simulink model "w3_warplab_agc"  (Simulink 7.7)
settings: Solver=ode45  StartTime=0.0  StopTime=1e4  RelTol=1e-3
PostLoadFcn:
  | w3_warplab_agc_init
InitFcn:
  | w3_warplab_agc_init
StartFcn:
  | w3_warplab_agc_init
undefined symbols (not defined in the file): gcbh, PHY_CONFIG_PKT_DET_CORR_THRESH, PHY_CONFIG_PKT_DET_ENERGY_THRESH, PHY_CONFIG_PKT_DET_MIN_DURR, xlBlockLoadCallback, xlGetNormalizedPeriod
libraries: xbsIndex_r4 x1039, xbsEDKLib_r4 x1, simulink x1
(part 1 of 7)
settings Model: Creator=murphpo  LastModifiedBy=mango
settings DebuggingCC: SolverPrmCheckMsg=none  InheritedTsInSrcMsg=none  FcnCallInpInsideContextMsg=Enable All  UnconnectedInputMsg=none  UnconnectedOutputMsg=none  UnconnectedLineMsg=none

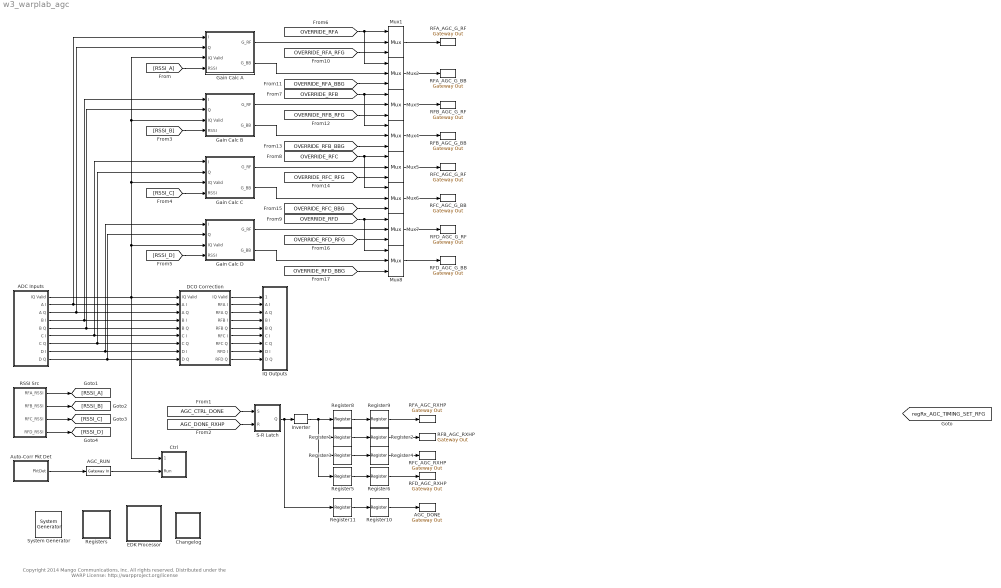
== system w3_warplab_agc ==
  note: Copyright 2014 Mango Communications, Inc. All rights reserved.
      |
      | Distributed under the WARP License:
      | http://warpproject.org/license
  " System Generator" : xbsIndex_r4/ System Generator  Tag=genX  SystemSampleTime=-1  xilinxfamily=virtex6  part=xc6vlx240t  speed=-2  package=ff1156  synthesis_tool=XST  clock_wrapper=Clock Enables  directory=./warplab_agc  proj_type=Project Navigator  Synth_file=XST Defaults  Impl_file=ISE Defaults  testbench=off  simulink_period=1  sysclk_period=10  dcm_input_clock_period=10  incr_netlist=off  trim_vbits=Everywhere in SubSystem  dbl_ovrd=According to Block Masks  core_generation=According to Block Masks  run_coregen=off  deprecated_control=off  eval_field=0  block_type=sysgen
  ADC Inputs : Subsystem
  AGC_DONE : xbsIndex_r4/Gateway Out  inherit_from_input=off  hdl_port=on  timing_constraint=None  locs_specified=off  LOCs={}  UseAsDAC=off  DACChannel='1'  block_type=gatewayout
  AGC_RUN : xbsIndex_r4/Gateway In  gui_display_data_type=Boolean  arith_type=Boolean  n_bits=16  bin_pt=14  preci_type=Single  exp_width=8  frac_width=24  quantization="Round  (unbiased: +/- Inf)"  overflow=Saturate  period=1  dbl_ovrd=off  timing_constraint=None  locs_specified=off  LOCs={}  UseAsADC=off  ADCChannel='1'  inherit_from_input=off  hdl_port=on  block_type=gatewayin
  Auto-Corr Pkt Det : Subsystem
  Changelog : Subsystem
  Ctrl : Subsystem
  DCO Correction : Subsystem
  EDK Processor : Subsystem  LoadFcn=xlBlockLoadCallback(gcbh);  mask(Xilinx EDK Processor Block){mode=EDK pcore generation, xmp=, MemVisToProc=<qt bgcolor="#FFFFFF"><div><img src="C:/Xilinx/14.4/ISE_DS/ISE/sysgen/data/images/registerplus.gif"> &lt;&lt;TIMING_RESET&gt;&gt;<br></div><div><img src="C:/Xilinx/14.4/ISE_DS/ISE/sysgen/data/images/registerplus.gif"> &lt;&lt;RSSI_PWR_CALIB&gt;&gt;<br></div><div><img src="C:/Xilinx/14.4/ISE_DS/ISE/sysgen/data/images/registerplus.gif"> &lt;&lt;IIR_COEF_B0&gt;&gt;<br></div><div><img src="C:/Xilinx/14.4/ISE_DS/ISE/sysgen/data/images/registerplus.gif"> &lt;&lt;IIR_COEF_A1&gt;&gt;<br></div><div><img src="C:/Xilinx/14.4/ISE_DS/ISE/sysgen/data/images/registerplus.gif"> &lt;&lt;RESET&gt;&gt;<br></div><div><img src="C:/Xilinx/14.4/ISE_DS/ISE/sysgen/data/images/registerplus.gif"> &lt;&lt;TIMING_AGC&gt;&gt;<br></div><div><img src="C:/Xilinx/14.4/ISE_DS/ISE/sysgen/data/images/registerplus.gif"> &lt;&lt;TARGET&gt;&gt;<br></div><div><img src="C:/Xilinx/14.4/ISE_DS/ISE/sysgen/data/images/registerplus.gif"> &lt;&lt;CONFIG&gt;&gt;<br></div><div><img src="C:/Xilinx/14.4/ISE_DS/ISE/sysgen/data/images/registerplus.gif"> &lt;&lt;RESET_MODE&gt;&gt;<br></div><div><img src="C:/Xilinx/14.4/ISE_DS/ISE/sysgen/data/images/registerplus.gif"> &lt;&lt;AGC_OVERRIDE&gt;&gt;<br></div><div><img src="C:/Xilinx/14.4/ISE_DS/ISE/sysgen/data/images/registerplus.gif"> &lt;&lt;RX_LENGTH&gt;&gt;<br></div><div><img src="C:/Xilinx/14.4/ISE_DS/ISE/sysgen/data/images/registerplus.gif"> &lt;&lt;TIMING_DCO&gt;&gt;<br></div></qt>, AvailableMemories=<empty>, portInterfaceTable={'exposed'=>[],'portdir'=>[],'portname'=>[],'shortname'=>[]}, bus_type_sgadvanced=, bus_type=AXI, baseaddr=0x80000000, baseaddr_lock_sgadvanced=, baseaddr_lock=off, dual_clock_sgadvanced=, dual_clock=on, reg_readback_sgadvanced=, reg_readback=on, ucf_file=, inheritDeviceType_sgadvanced=, inheritDeviceType=off, elf_file=, codebug_sgadvanced=, codebug=on, clock_name=plb, internalPortList={}, resetPolarity=0, memxtable={'mladdr'=>[0.00000000000000000,1.00000000000000000,2.00000000000000000,3.00000000000000000,4.00000000000000000,5.00000000000000000,6.00000000000000000,7.00000000000000000,8.00000000000000000,9.00000000000000000,10.00000000000000000,11.00000000000000000],'mlist'=>['w3_warplab_agc/Registers/From Register9','w3_warplab_agc/Registers/From Register8','w3_warplab_agc/Registers/From Register7','w3_warplab_agc/Registers/From Register6','w3_warplab_agc/Registers/From Register5','w3_warplab_agc/Registers/From Register4','w3_warplab_agc/Registers/From Register3','w3_warplab_agc/Registers/From Register2','w3_warplab_agc/Registers/From Register12','w3_warplab_agc/Registers/From Register11','w3_warplab_agc/Registers/From Register10','w3_warplab_agc/Registers/From Register1'],'mlname'=>['\\'TIMING_RESET\\'','\\'RSSI_PWR_CALIB\\'','\\'IIR_COEF_B0\\'','\\'IIR_COEF_A1\\'','\\'RESET\\'','\\'TIMING_AGC\\'','\\'TARGET\\'','\\'CONFIG\\'','\\'RESET_MODE\\'','\\'AGC_OVERRIDE\\'','\\'RX_LENGTH\\'','\\'TIMING_DCO\\''],'mlstate'=>[0.00000000000000000,0.00000000000000000,0.00000000000000000,0.00000000000000000,0.00000000000000000,0.00000000000000000,0.00000000000000000,0.00000000000000000,0.00000000000000000,0.00000000000000000,0.00000000000000000,0.00000000000000000]}, procinfo={}, memmapdirty=off, blockname=, xpsintstyle=default, has_advanced_control=0, sggui_pos=-1,-1,-1,-1, block_type=edkprocessor, block_version=2.7, sg_icon_stat=62,64,-1,-1,white,blue,0,07734,right,,[ ],[ ], sg_mask_display=|, sg_list_contents={'table'=>{'AvailableMemories'=>'popup(<empty>)'}}, sg_blockgui_xml=}
      mask sg_mask_display=|
      | fprintf('','COMMENT: begin icon graphics');
      | patch([0 62 62 0 0 ],[0 0 64 64 0 ],[0.77 0.82 0.91 ]);
      | plot([0 62 62 0 0 ],[0 0 64 64 0 ]);
      | patch([13.2 24.76 32.76 40.76 48.76 32.76 21.2 13.2 ],[40.88 40.88 48.88 40.88 48.88 48.88 48.88 40.88 ],[1 1 1 ]);
      | patch([21.2 32.76 24.76 13.2 21.2 ],[32.88 32.88 40.88 40.88 32.88 ],[0.931 0.946 0.973 ]);
      | patch([13.2 24.76 32.76 21.2 13.2 ],[24.88 24.88 32.88 32.88 24.88 ],[1 1 1 ]);
      | patch([21.2 48.76 40.76 32.76 24.76 13.2 21.2 ],[16.88 16.88 24.88 16.88 24.88 24.88 16.88 ],[0.931 0.946 0.973 ]);
      | fprintf('','COMMENT: end icon graphics');
      | fprintf('','COMMENT: begin icon text');
      | fprintf('','COMMENT: end icon text');
      mask prompts: mode "Configure Processor for"; xmp "XPS Project"; MemVisToProc ""; AvailableMemories "Available Memories"; portInterfaceTable ""; bus_type_sgadvanced ""; bus_type "Bus Type"; baseaddr "Base Address"; baseaddr_lock_sgadvanced ""; baseaddr_lock "Lock"; dual_clock_sgadvanced ""; dual_clock "Dual Clocks"; reg_readback_sgadvanced ""; reg_readback "Register Read-Back"; ucf_file "Constraint File"; inheritDeviceType_sgadvanced ""; inheritDeviceType "Inherit Device Type"; elf_file "Initial Program"; codebug_sgadvanced ""; codebug "Enable Co-Debug with Xilinx SDK (Beta)"; clock_name ""; internalPortList ""; resetPolarity ""; memxtable ""; procinfo ""; memmapdirty ""; blockname ""; xpsintstyle ""; has_advanced_control ""; sggui_pos ""; block_type ""; block_version ""; sg_icon_stat ""; sg_mask_display ""; sg_list_contents ""; sg_blockgui_xml ""
      mask help: Xilinx EDK Processor
      mask init:
      | try
      |   tmp_gcb = gcb;
      |   tmp_gcbh = gcbh;
      |   if (strcmp('SysGenIndex',get_param(bdroot(tmp_gcbh),'tag')) && ~isempty(regexp(bdroot(tmp_gcb), '^xbs', 'once')))
      |     return;
      |   end;
      |   xlMungeMaskParams;
      | 
      |   block_type='edkprocessor';
      | 
      |   serialized_declarations = '{''block_type''=>''String''}';
      |   xledkprocessor_init();
      |   ptable_ = xlblockprep(get_param(tmp_gcb, 'MaskWSVariables'));
      |   try
      |     xlBlockMoveCallback(tmp_gcbh);
      |   catch 
      |      clear global xl_updateicon_recursion_guard;
      |   end;
      | catch
      |   global dbgsysgen;
      |   if(~isempty(dbgsysgen) && dbgsysgen)
      |     e = regexprep(lasterr, '\n', '\nError: ');
      |     disp(['Error: While running MaskInit code on block ' tmp_gcb ': ' e]);
      |     error(e);
      |   end
      | end
      settings: CopyFcn=xlProcBlockCopyCallback(gcbh);xlBlockMoveCallback(gcbh);  DeleteFcn=xlDestroyGui(gcbh);  ModelCloseFcn=xlDestroyGui(gcbh);  PreSaveFcn=xlBlockPreSaveCallback(gcbh);  PostSaveFcn=xlBlockPostSaveCallback(gcbh);  DestroyFcn=xlDestroyGui(gcbh);  OpenFcn=bh=gcbh;xlProcBlockCallbacks('populatesharedmemorylistbox',bh);xlOpenGui(bh, 'edkprocessor_gui.xml', @xlProcBlockEnablement, @xlProcBlockAction);  CloseFcn=xlDestroyGui(gcbh);  MoveFcn=xlBlockMoveCallback(gcbh);
      mask Help: eval('');xlDoc('-book','sysgen','-topic','EDK_Processor');
      mask StyleString: popup(EDK pcore generation|HDL netlisting),edit,edit,edit,edit,edit,popup(AXI|PLB),edit,edit,checkbox,edit,checkbox,edit,checkbox,edit,edit,checkbox,edit,edit,checkbox,edit,edit,edit,edit,edit,edit,edit,edit,edit,edit,edit,edit,edit,edit,edit,edit
      mask Display:
      | fprintf('','COMMENT: begin icon graphics');
      | patch([0 62 62 0 0 ],[0 0 64 64 0 ],[0.77 0.82 0.91 ]);
      | plot([0 62 62 0 0 ],[0 0 64 64 0 ]);
      | patch([13.2 24.76 32.76 40.76 48.76 32.76 21.2 13.2 ],[40.88 40.88 48.88 40.88 48.88 48.88 48.88 40.88 ],[1 1 1 ]);
      | patch([21.2 32.76 24.76 13.2 21.2 ],[32.88 32.88 40.88 40.88 32.88 ],[0.931 0.946 0.973 ]);
      | patch([13.2 24.76 32.76 21.2 13.2 ],[24.88 24.88 32.88 32.88 24.88 ],[1 1 1 ]);
      | patch([21.2 48.76 40.76 32.76 24.76 13.2 21.2 ],[16.88 16.88 24.88 16.88 24.88 24.88 16.88 ],[0.931 0.946 0.973 ]);
      | fprintf('','COMMENT: end icon graphics');
      | fprintf('','COMMENT: begin icon text');
      | disp('');
      | 
      | fprintf('','COMMENT: end icon text');
  Gain Calc A : Subsystem
  Gain Calc B : Subsystem
  Gain Calc C : Subsystem
  Gain Calc D : Subsystem
  IQ Outputs : Subsystem
  Inverter : xbsIndex_r4/Inverter  en=off  latency=0  dbl_ovrd=off  block_type=inv
      settings: xl_area=[0 0 0 0 0 0 0]  block_version=VER_STRING_GOES_HERE
  Mux{1..8} (8 alike) : xbsIndex_r4/Mux  inputs=2  en=off  latency=0  precision=Full  arith_type=Unsigned  n_bits=16  bin_pt=14  quantization=Truncate  overflow=Wrap  dbl_ovrd=off  block_type=mux
  RFA_AGC_G_BB : xbsIndex_r4/Gateway Out  inherit_from_input=off  hdl_port=on  timing_constraint=None  locs_specified=off  LOCs={}  UseAsDAC=off  DACChannel='1'  block_type=gatewayout
  RFA_AGC_G_RF : xbsIndex_r4/Gateway Out  inherit_from_input=off  hdl_port=on  timing_constraint=None  locs_specified=off  LOCs={}  UseAsDAC=off  DACChannel='1'  block_type=gatewayout
  RFA_AGC_RXHP : xbsIndex_r4/Gateway Out  inherit_from_input=off  hdl_port=on  timing_constraint=None  locs_specified=off  LOCs={}  UseAsDAC=off  DACChannel='1'  block_type=gatewayout
  RFB_AGC_G_BB : xbsIndex_r4/Gateway Out  inherit_from_input=off  hdl_port=on  timing_constraint=None  locs_specified=off  LOCs={}  UseAsDAC=off  DACChannel='1'  block_type=gatewayout
  RFB_AGC_G_RF : xbsIndex_r4/Gateway Out  inherit_from_input=off  hdl_port=on  timing_constraint=None  locs_specified=off  LOCs={}  UseAsDAC=off  DACChannel='1'  block_type=gatewayout
  RFB_AGC_RXHP : xbsIndex_r4/Gateway Out  inherit_from_input=off  hdl_port=on  timing_constraint=None  locs_specified=off  LOCs={}  UseAsDAC=off  DACChannel='1'  block_type=gatewayout
  RFC_AGC_G_BB : xbsIndex_r4/Gateway Out  inherit_from_input=off  hdl_port=on  timing_constraint=None  locs_specified=off  LOCs={}  UseAsDAC=off  DACChannel='1'  block_type=gatewayout
  RFC_AGC_G_RF : xbsIndex_r4/Gateway Out  inherit_from_input=off  hdl_port=on  timing_constraint=None  locs_specified=off  LOCs={}  UseAsDAC=off  DACChannel='1'  block_type=gatewayout
  RFC_AGC_RXHP : xbsIndex_r4/Gateway Out  inherit_from_input=off  hdl_port=on  timing_constraint=None  locs_specified=off  LOCs={}  UseAsDAC=off  DACChannel='1'  block_type=gatewayout
  RFD_AGC_G_BB : xbsIndex_r4/Gateway Out  inherit_from_input=off  hdl_port=on  timing_constraint=None  locs_specified=off  LOCs={}  UseAsDAC=off  DACChannel='1'  block_type=gatewayout
  RFD_AGC_G_RF : xbsIndex_r4/Gateway Out  inherit_from_input=off  hdl_port=on  timing_constraint=None  locs_specified=off  LOCs={}  UseAsDAC=off  DACChannel='1'  block_type=gatewayout
  RFD_AGC_RXHP : xbsIndex_r4/Gateway Out  inherit_from_input=off  hdl_port=on  timing_constraint=None  locs_specified=off  LOCs={}  UseAsDAC=off  DACChannel='1'  block_type=gatewayout
  RSSI Src : Subsystem
  Register{1..6,8..11} (10 alike) : xbsIndex_r4/Register  init=0  rst=off  en=off  dbl_ovrd=off  block_type=register
  Registers : Subsystem
  S-R Latch : Subsystem
  tag scope: regRx_AGC_TIMING_SET_RFG=global
  wires:
  AGC_RUN/1 -> Ctrl/2(Run)
  [AGC_CTRL_DONE] -> S-R Latch/1(S)
  [AGC_DONE_RXHP] -> S-R Latch/2(R)
  S-R Latch/1(Q) -> Inverter/1, Register11/1
  Register8/1 -> Register9/1
  Register9/1 -> RFA_AGC_RXHP/1
  Inverter/1 -> Register8/1, Register1/1, Register3/1, Register5/1
  Register10/1 -> AGC_DONE/1
  Register11/1 -> Register10/1
  Register1/1 -> Register2/1
  Register2/1 -> RFB_AGC_RXHP/1
  ADC Inputs/1(IQ Valid) -> DCO Correction/1(IQ Valid), Gain Calc A/3(IQ Valid), Gain Calc B/3(IQ Valid), Gain Calc C/3(IQ Valid), Gain Calc D/3(IQ Valid), Ctrl/1(IQ Valid)
  ADC Inputs/2(A I) -> DCO Correction/2(A I), Gain Calc A/1(I)
  ADC Inputs/3(A Q) -> DCO Correction/3(A Q), Gain Calc A/2(Q)
  ADC Inputs/4(B I) -> DCO Correction/4(B I), Gain Calc B/1(I)
  ADC Inputs/5(B Q) -> DCO Correction/5(B Q), Gain Calc B/2(Q)
  ADC Inputs/6(C I) -> DCO Correction/6(C I), Gain Calc C/1(I)
  ADC Inputs/7(C Q) -> DCO Correction/7(C Q), Gain Calc C/2(Q)
  ADC Inputs/8(D I) -> DCO Correction/8(D I), Gain Calc D/1(I)
  ADC Inputs/9(D Q) -> DCO Correction/9(D Q), Gain Calc D/2(Q)
  DCO Correction/1(" IQ Valid") -> IQ Outputs/1(IQ Valid)
  DCO Correction/2(" RFA I") -> IQ Outputs/2(A I)
  DCO Correction/3(" RFA Q") -> IQ Outputs/3(A Q)
  DCO Correction/4(RFB I) -> IQ Outputs/4(B I)
  DCO Correction/5(RFB Q) -> IQ Outputs/5(B Q)
  DCO Correction/6(RFC I) -> IQ Outputs/6(C I)
  DCO Correction/7(RFC Q) -> IQ Outputs/7(C Q)
  DCO Correction/8(RFD I) -> IQ Outputs/8(D I)
  DCO Correction/9(RFD Q) -> IQ Outputs/9(D Q)
  RSSI Src/1(" RFA_RSSI") -> [RSSI_A]
  RSSI Src/2(" RFB_RSSI") -> [RSSI_B]
  [RSSI_A] -> Gain Calc A/4(RSSI)
  [RSSI_B] -> Gain Calc B/4(RSSI)
  [RSSI_C] -> Gain Calc C/4(RSSI)
  [RSSI_D] -> Gain Calc D/4(RSSI)
  Register3/1 -> Register4/1
  Register4/1 -> RFC_AGC_RXHP/1
  Register5/1 -> Register6/1
  Register6/1 -> RFD_AGC_RXHP/1
  RSSI Src/3(" RFC_RSSI") -> [RSSI_C]
  RSSI Src/4(" RFD_RSSI") -> [RSSI_D]
  [OVERRIDE_RFA] -> Mux1/1, Mux2/1
  Mux1/1 -> RFA_AGC_G_RF/1
  Mux2/1 -> RFA_AGC_G_BB/1
  Mux3/1 -> RFB_AGC_G_RF/1
  Mux4/1 -> RFB_AGC_G_BB/1
  Mux5/1 -> RFC_AGC_G_RF/1
  Mux6/1 -> RFC_AGC_G_BB/1
  Mux7/1 -> RFD_AGC_G_RF/1
  Mux8/1 -> RFD_AGC_G_BB/1
  [OVERRIDE_RFB] -> Mux3/1, Mux4/1
  [OVERRIDE_RFA_RFG] -> Mux1/3
  [OVERRIDE_RFA_BBG] -> Mux2/3
  Gain Calc A/1(G_RF) -> Mux1/2
  Gain Calc A/2(G_BB) -> Mux2/2
  Gain Calc B/1(G_RF) -> Mux3/2
  [OVERRIDE_RFB_RFG] -> Mux3/3
  Gain Calc B/2(G_BB) -> Mux4/2
  [OVERRIDE_RFB_BBG] -> Mux4/3
  [OVERRIDE_RFC] -> Mux5/1, Mux6/1
  [OVERRIDE_RFD] -> Mux7/1, Mux8/1
  Gain Calc C/1(G_RF) -> Mux5/2
  Gain Calc C/2(G_BB) -> Mux6/2
  Gain Calc D/1(G_RF) -> Mux7/2
  Gain Calc D/2(G_BB) -> Mux8/2
  [OVERRIDE_RFC_RFG] -> Mux5/3
  [OVERRIDE_RFC_BBG] -> Mux6/3
  [OVERRIDE_RFD_RFG] -> Mux7/3
  [OVERRIDE_RFD_BBG] -> Mux8/3
  Auto-Corr Pkt Det/1(PktDet) -> AGC_RUN/1

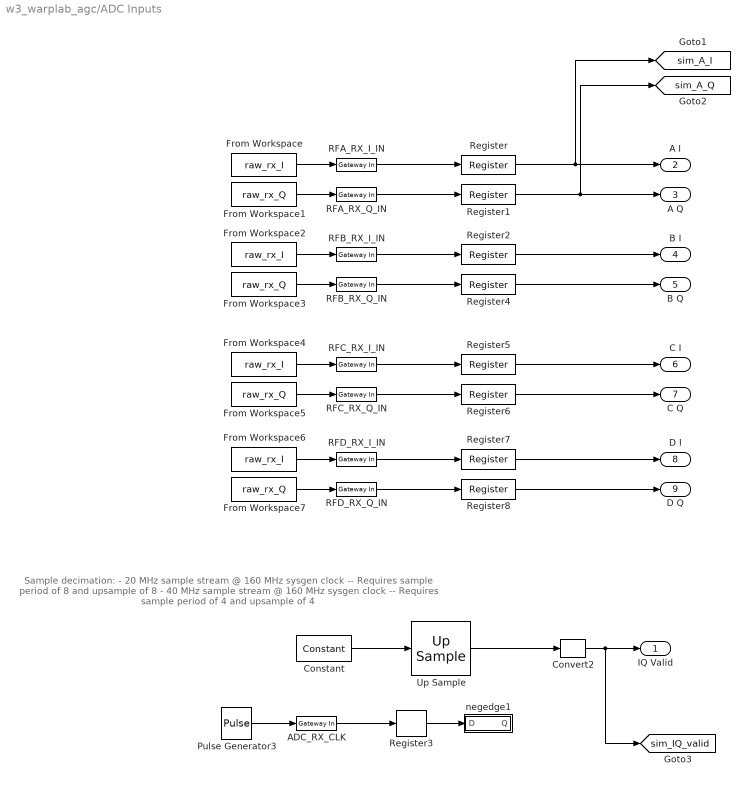
== system w3_warplab_agc/ADC Inputs ==
  note: Sample decimation:
      |   - 20 MHz sample stream @ 160 MHz sysgen clock -- Requires sample period of 8 and upsample of 8
      |   - 40 MHz sample stream @ 160 MHz sysgen clock -- Requires sample period of 4 and upsample of 4
  ADC_RX_CLK : xbsIndex_r4/Gateway In  gui_display_data_type=Boolean  arith_type=Boolean  n_bits=1  bin_pt=0  preci_type=Single  exp_width=8  frac_width=24  quantization="Round  (unbiased: +/- Inf)"  overflow=Saturate  period=1  dbl_ovrd=off  timing_constraint=None  locs_specified=off  LOCs={}  UseAsADC=off  ADCChannel='1'  inherit_from_input=off  hdl_port=on  block_type=gatewayin
  Constant : xbsIndex_r4/Constant  const=1  gui_display_data_type=Boolean  arith_type=Boolean  n_bits=16  bin_pt=14  preci_type=Single  exp_width=8  frac_width=24  explicit_period=on  period=4  equ=P=C  opselect=C  inp2=PCIN>>17  opr=+  inp1=P  carry=CIN  dbl_ovrd=off  block_type=constant
  Convert2 : xbsIndex_r4/Convert  gui_display_data_type=Boolean  arith_type=Boolean  n_bits=1  bin_pt=0  float_type=Single  exp_bits=8  fraction_bits=24  quantization=Truncate  overflow=Wrap  en=off  latency=0  dbl_ovrd=off  pipeline=off  block_type=convert
  From Workspace{,2,4,6} (4 alike) : FromWorkspace  VariableName=raw_rx_I  SampleTime=4  Interpolate=off  OutputAfterFinalValue=Setting to zero
  From Workspace{1,3,5,7} (4 alike) : FromWorkspace  VariableName=raw_rx_Q  SampleTime=4  Interpolate=off  OutputAfterFinalValue=Setting to zero
  Pulse Generator3 : DiscretePulseGenerator  Period=8  PulseWidth=4
  RFA_RX_I_IN : xbsIndex_r4/Gateway In  gui_display_data_type=Fixed-point  arith_type="Signed  (2's comp)"  n_bits=12  bin_pt=11  preci_type=Single  exp_width=8  frac_width=24  quantization="Round  (unbiased: +/- Inf)"  overflow=Saturate  period=1  dbl_ovrd=off  timing_constraint=None  locs_specified=off  LOCs={}  UseAsADC=off  ADCChannel='1'  inherit_from_input=off  hdl_port=on  block_type=gatewayin
  RFA_RX_Q_IN : xbsIndex_r4/Gateway In  gui_display_data_type=Fixed-point  arith_type="Signed  (2's comp)"  n_bits=12  bin_pt=11  preci_type=Single  exp_width=8  frac_width=24  quantization="Round  (unbiased: +/- Inf)"  overflow=Saturate  period=1  dbl_ovrd=off  timing_constraint=None  locs_specified=off  LOCs={}  UseAsADC=off  ADCChannel='1'  inherit_from_input=off  hdl_port=on  block_type=gatewayin
  RFB_RX_I_IN : xbsIndex_r4/Gateway In  gui_display_data_type=Fixed-point  arith_type="Signed  (2's comp)"  n_bits=12  bin_pt=11  preci_type=Single  exp_width=8  frac_width=24  quantization="Round  (unbiased: +/- Inf)"  overflow=Saturate  period=1  dbl_ovrd=off  timing_constraint=None  locs_specified=off  LOCs={}  UseAsADC=off  ADCChannel='1'  inherit_from_input=off  hdl_port=on  block_type=gatewayin
  RFB_RX_Q_IN : xbsIndex_r4/Gateway In  gui_display_data_type=Fixed-point  arith_type="Signed  (2's comp)"  n_bits=12  bin_pt=11  preci_type=Single  exp_width=8  frac_width=24  quantization="Round  (unbiased: +/- Inf)"  overflow=Saturate  period=1  dbl_ovrd=off  timing_constraint=None  locs_specified=off  LOCs={}  UseAsADC=off  ADCChannel='1'  inherit_from_input=off  hdl_port=on  block_type=gatewayin
  RFC_RX_I_IN : xbsIndex_r4/Gateway In  gui_display_data_type=Fixed-point  arith_type="Signed  (2's comp)"  n_bits=12  bin_pt=11  preci_type=Single  exp_width=8  frac_width=24  quantization="Round  (unbiased: +/- Inf)"  overflow=Saturate  period=1  dbl_ovrd=off  timing_constraint=None  locs_specified=off  LOCs={}  UseAsADC=off  ADCChannel='1'  inherit_from_input=off  hdl_port=on  block_type=gatewayin
  RFC_RX_Q_IN : xbsIndex_r4/Gateway In  gui_display_data_type=Fixed-point  arith_type="Signed  (2's comp)"  n_bits=12  bin_pt=11  preci_type=Single  exp_width=8  frac_width=24  quantization="Round  (unbiased: +/- Inf)"  overflow=Saturate  period=1  dbl_ovrd=off  timing_constraint=None  locs_specified=off  LOCs={}  UseAsADC=off  ADCChannel='1'  inherit_from_input=off  hdl_port=on  block_type=gatewayin
  RFD_RX_I_IN : xbsIndex_r4/Gateway In  gui_display_data_type=Fixed-point  arith_type="Signed  (2's comp)"  n_bits=12  bin_pt=11  preci_type=Single  exp_width=8  frac_width=24  quantization="Round  (unbiased: +/- Inf)"  overflow=Saturate  period=1  dbl_ovrd=off  timing_constraint=None  locs_specified=off  LOCs={}  UseAsADC=off  ADCChannel='1'  inherit_from_input=off  hdl_port=on  block_type=gatewayin
  RFD_RX_Q_IN : xbsIndex_r4/Gateway In  gui_display_data_type=Fixed-point  arith_type="Signed  (2's comp)"  n_bits=12  bin_pt=11  preci_type=Single  exp_width=8  frac_width=24  quantization="Round  (unbiased: +/- Inf)"  overflow=Saturate  period=1  dbl_ovrd=off  timing_constraint=None  locs_specified=off  LOCs={}  UseAsADC=off  ADCChannel='1'  inherit_from_input=off  hdl_port=on  block_type=gatewayin
  Register{,1..8} (9 alike) : xbsIndex_r4/Register  init=0  rst=off  en=off  dbl_ovrd=off  block_type=register
  Up Sample : xbsIndex_r4/Up Sample  sample_ratio=4  copy_samples=off  en=off  latency=0  dbl_ovrd=off  block_type=usamp
  negedge1 : Subsystem
  IQ Valid : Outport
  A I : Outport  Port=2
  A Q : Outport  Port=3
  B I : Outport  Port=4
  B Q : Outport  Port=5
  C I : Outport  Port=6
  C Q : Outport  Port=7
  D I : Outport  Port=8
  D Q : Outport  Port=9
  tag scope: sim_A_I=global, sim_A_Q=global, sim_IQ_valid=global
  wires:
  From Workspace/1 -> RFA_RX_I_IN/1
  From Workspace1/1 -> RFA_RX_Q_IN/1
  RFA_RX_I_IN/1 -> Register/1
  RFA_RX_Q_IN/1 -> Register1/1
  From Workspace2/1 -> RFB_RX_I_IN/1
  From Workspace3/1 -> RFB_RX_Q_IN/1
  RFB_RX_I_IN/1 -> Register2/1
  RFB_RX_Q_IN/1 -> Register4/1
  Up Sample/1 -> Convert2/1
  Register3/1 -> negedge1/1(D)
  ADC_RX_CLK/1 -> Register3/1
  Pulse Generator3/1 -> ADC_RX_CLK/1
  Convert2/1 -> IQ Valid/1, [sim_IQ_valid]
  RFC_RX_I_IN/1 -> Register5/1
  RFC_RX_Q_IN/1 -> Register6/1
  RFD_RX_I_IN/1 -> Register7/1
  RFD_RX_Q_IN/1 -> Register8/1
  Constant/1 -> Up Sample/1
  From Workspace4/1 -> RFC_RX_I_IN/1
  From Workspace5/1 -> RFC_RX_Q_IN/1
  From Workspace6/1 -> RFD_RX_I_IN/1
  From Workspace7/1 -> RFD_RX_Q_IN/1
  Register/1 -> A I/1, [sim_A_I]
  Register1/1 -> A Q/1, [sim_A_Q]
  Register2/1 -> B I/1
  Register4/1 -> B Q/1
  Register5/1 -> C I/1
  Register6/1 -> C Q/1
  Register7/1 -> D I/1
  Register8/1 -> D Q/1

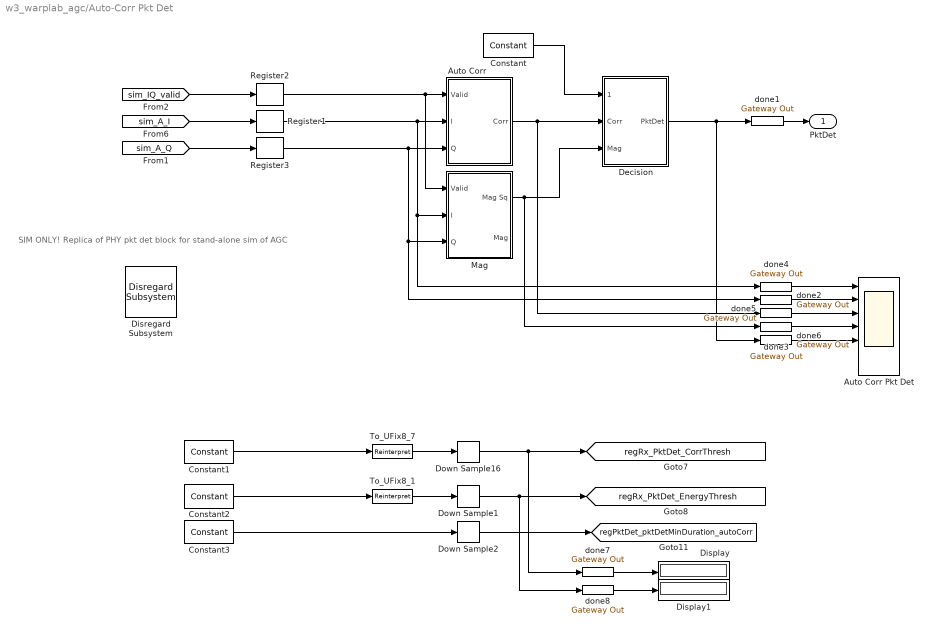
== system w3_warplab_agc/Auto-Corr Pkt Det ==
  note: SIM ONLY!
      | Replica of PHY pkt det block
      | for stand-alone sim of AGC
  Auto Corr : Subsystem
  Auto Corr Pkt Det : Scope  NumInputPorts=7
      settings: TimeRange=10000  YMin=-0.4~-0.4~-0.2~-0.2~-0.01~-1~0  YMax=0.4~0.4~0.2~0.2~0.02~1~0.8  SaveName=ScopeData28
  Constant : xbsIndex_r4/Constant  const=0  gui_display_data_type=Boolean  arith_type=Boolean  n_bits=16  bin_pt=14  preci_type=Single  exp_width=8  frac_width=24  explicit_period=off  period=1  equ=P=C  opselect=C  inp2=PCIN>>17  opr=+  inp1=P  carry=CIN  dbl_ovrd=off  block_type=constant
  Constant1 : xbsIndex_r4/Constant  const=PHY_CONFIG_PKT_DET_CORR_THRESH  gui_display_data_type=Fixed-point  arith_type=Unsigned  n_bits=8  bin_pt=0  preci_type=Single  exp_width=8  frac_width=24  explicit_period=on  period=1  equ=P=C  opselect=C  inp2=PCIN>>17  opr=+  inp1=P  carry=CIN  dbl_ovrd=off  block_type=constant
  Constant2 : xbsIndex_r4/Constant  const=PHY_CONFIG_PKT_DET_ENERGY_THRESH  gui_display_data_type=Fixed-point  arith_type=Unsigned  n_bits=16  bin_pt=0  preci_type=Single  exp_width=8  frac_width=24  explicit_period=on  period=1  equ=P=C  opselect=C  inp2=PCIN>>17  opr=+  inp1=P  carry=CIN  dbl_ovrd=off  block_type=constant
  Constant3 : xbsIndex_r4/Constant  const=PHY_CONFIG_PKT_DET_MIN_DURR  gui_display_data_type=Fixed-point  arith_type=Unsigned  n_bits=6  bin_pt=0  preci_type=Single  exp_width=8  frac_width=24  explicit_period=on  period=1  equ=P=C  opselect=C  inp2=PCIN>>17  opr=+  inp1=P  carry=CIN  dbl_ovrd=off  block_type=constant
  Decision : Subsystem
  Display : Display
  Display1 : Display
  Disregard Subsystem : xbsIndex_r4/Disregard Subsystem  Tag=discardX  block_type=disregard
  Down Sample1 : xbsIndex_r4/Down Sample  sample_ratio=8  sample_phase="Last Value of Frame  (most efficient)"  en=off  latency=1  dbl_ovrd=off  block_type=dsamp
      settings: block_version=VER_STRING_GOES_HERE
  Down Sample16 : xbsIndex_r4/Down Sample  sample_ratio=8  sample_phase="Last Value of Frame  (most efficient)"  en=off  latency=1  dbl_ovrd=off  block_type=dsamp
      settings: block_version=VER_STRING_GOES_HERE
  Down Sample2 : xbsIndex_r4/Down Sample  sample_ratio=8  sample_phase="Last Value of Frame  (most efficient)"  en=off  latency=1  dbl_ovrd=off  block_type=dsamp
      settings: block_version=VER_STRING_GOES_HERE
  Mag : Subsystem
  Register1 : xbsIndex_r4/Register  init=0  rst=off  en=off  dbl_ovrd=off  block_type=register
  Register2 : xbsIndex_r4/Register  init=0  rst=off  en=off  dbl_ovrd=off  block_type=register
  Register3 : xbsIndex_r4/Register  init=0  rst=off  en=off  dbl_ovrd=off  block_type=register
  To_UFix8_1 : xbsIndex_r4/Reinterpret  force_arith_type=on  arith_type=Unsigned  force_bin_pt=on  bin_pt=8  block_type=cast
      settings: infoedit="Changes type of samples without altering their binary representation.<P><P>Hardware notes: In hardware this block costs nothing.<P><P>Example:  Suppose the input is 6 bits wide, signed, with 2 fractional bits, and the output is forced to unsigned with 0 fractional bits.  Then an input of -2.0 (1110.00 in binary 2's complement) becomes an output of 56 (111000 in binary)."  block_version=VER_STRING_GOES_HERE
  To_UFix8_7 : xbsIndex_r4/Reinterpret  force_arith_type=on  arith_type=Unsigned  force_bin_pt=on  bin_pt=7  block_type=cast
      settings: infoedit="Changes type of samples without altering their binary representation.<P><P>Hardware notes: In hardware this block costs nothing.<P><P>Example:  Suppose the input is 6 bits wide, signed, with 2 fractional bits, and the output is forced to unsigned with 0 fractional bits.  Then an input of -2.0 (1110.00 in binary 2's complement) becomes an output of 56 (111000 in binary)."  block_version=VER_STRING_GOES_HERE
  done{1..8} (8 alike) : xbsIndex_r4/Gateway Out  inherit_from_input=off  hdl_port=off  timing_constraint=None  locs_specified=off  LOCs={}  UseAsDAC=off  DACChannel='1'  block_type=gatewayout
      settings: infoedit="Gateway out block.  Converts Xilinx fixed point inputs into ouputs of type Simulink integer, double, or fixed point.<P><P>Hardware notes:  In hardware these blocks become top level output ports or are discarded, depending on how they are configured."  xl_area=[0 0 0 0 1 0 0]  block_version=VER_STRING_GOES_HERE
  PktDet : Outport
  tag scope: regPktDet_pktDetMinDuration_autoCorr=global, regRx_PktDet_CorrThresh=global, regRx_PktDet_EnergyThresh=global
  wires:
  done4/1 -> Auto Corr Pkt Det/1
  [sim_A_Q] -> Register3/1
  [sim_A_I] -> Register1/1
  [sim_IQ_valid] -> Register2/1
  done2/1 -> Auto Corr Pkt Det/2
  done6/1 -> Auto Corr Pkt Det/5
  Register1/1 -> Auto Corr/2(I), Mag/2(I), done4/1
  Register3/1 -> Auto Corr/3(Q), Mag/3(Q), done2/1
  Register2/1 -> Auto Corr/1(Valid), Mag/1(Valid)
  Auto Corr/1(Corr) -> Decision/2(Corr), done5/1
  Mag/1(Mag Sq) -> Decision/3(Mag), done3/1
  done5/1 -> Auto Corr Pkt Det/3
  done3/1 -> Auto Corr Pkt Det/4
  Decision/1(PktDet) -> done6/1, done1/1
  Constant/1 -> Decision/1(PktDet Reset)
  done1/1 -> PktDet/1
  To_UFix8_7/1 -> Down Sample16/1
  To_UFix8_1/1 -> Down Sample1/1
  Down Sample16/1 -> [regRx_PktDet_CorrThresh], done7/1
  Down Sample1/1 -> [regRx_PktDet_EnergyThresh], done8/1
  Constant3/1 -> Down Sample2/1
  Down Sample2/1 -> [regPktDet_pktDetMinDuration_autoCorr]
  Constant1/1 -> To_UFix8_7/1
  Constant2/1 -> To_UFix8_1/1
  done7/1 -> Display/1
  done8/1 -> Display1/1

== system w3_warplab_agc/Changelog ==
  note: 3.00.a:
      | - Initial release.  Modified from 802.11 Reference Design
  note: 3.01.a:
      | - Fixed bug in handover between DCO and IIR HPF outputs.

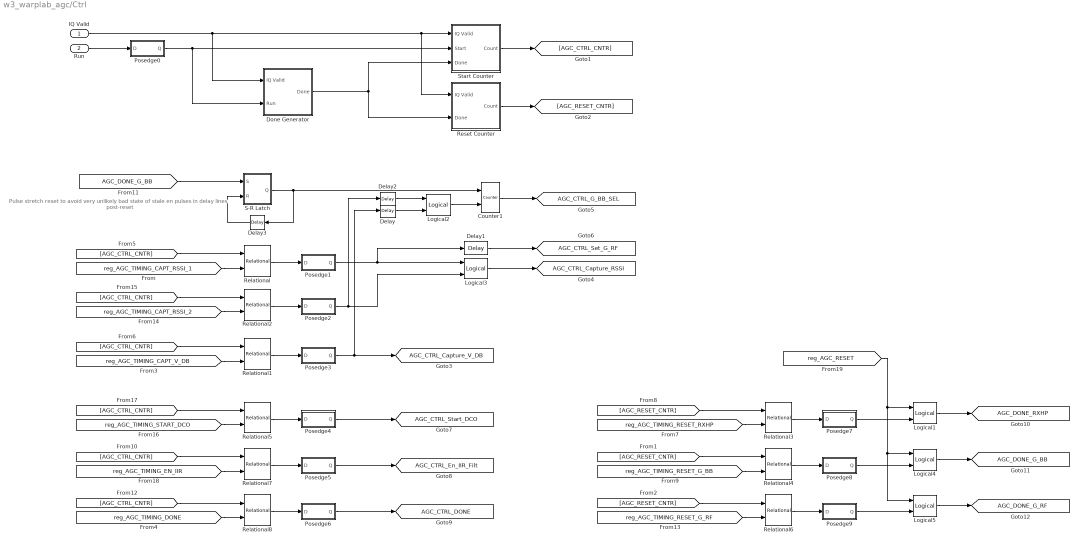
== system w3_warplab_agc/Ctrl ==
  note: Pulse stretch reset to avoid very
      | unlikely bad state of stale
      | en pulses in delay lines
      | post-reset
  IQ Valid : Inport
  Run : Inport  Port=2
  Counter1 : xbsIndex_r4/Counter  cnt_type=Free Running  cnt_to=1023  operation=Up  start_count=0  cnt_by_val=1  arith_type=Unsigned  n_bits=2  bin_pt=0  load_pin=off  rst=on  en=on  explicit_period=off  period=1  dbl_ovrd=off  use_behavioral_HDL=off  implementation=Fabric  block_type=counter
  Delay : xbsIndex_r4/Delay  rst=off  infoeditControl=Selection of Reset will increase slice count due to use of real FFs and instead of SRLs  en=off  latency=2  dbl_ovrd=off  reg_retiming=off  block_type=delay
      settings: xl_area=[7 14 0 14 0 0 0]  block_version=VER_STRING_GOES_HERE
  Delay1 : xbsIndex_r4/Delay  rst=off  infoeditControl=Selection of Reset will increase slice count due to use of real FFs and instead of SRLs  en=off  latency=5  dbl_ovrd=off  reg_retiming=off  block_type=delay
      settings: xl_area=[7 14 0 14 0 0 0]  block_version=VER_STRING_GOES_HERE
  Delay2 : xbsIndex_r4/Delay  rst=off  infoeditControl=Selection of Reset will increase slice count due to use of real FFs and instead of SRLs  en=off  latency=6  dbl_ovrd=off  reg_retiming=off  block_type=delay
      settings: xl_area=[7 14 0 14 0 0 0]  block_version=VER_STRING_GOES_HERE
  Delay3 : xbsIndex_r4/Delay  rst=off  infoeditControl=Selection of Reset will increase slice count due to use of real FFs and instead of SRLs  en=off  latency=6  dbl_ovrd=off  reg_retiming=off  block_type=delay
      settings: xl_area=[7 14 0 14 0 0 0]  block_version=VER_STRING_GOES_HERE
  Done Generator : Subsystem
  Logical{1..5} (5 alike) : xbsIndex_r4/Logical  logical_function=OR  inputs=2  en=off  latency=0  precision=Full  arith_type=Unsigned  n_bits=16  bin_pt=0  align_bp=on  dbl_ovrd=off  block_type=logical
  Posedge0 : Subsystem
  Posedge1 : Subsystem
  Posedge2 : Subsystem
  Posedge3 : Subsystem
  Posedge4 : Subsystem
  Posedge5 : Subsystem
  Posedge6 : Subsystem
  Posedge7 : Subsystem
  Posedge8 : Subsystem
  Posedge9 : Subsystem
  Relational{,1..8} (9 alike) : xbsIndex_r4/Relational  mode=a>=b  en=off  latency=0  dbl_ovrd=off  block_type=relational
  Reset Counter : Subsystem
  S-R Latch : Subsystem
  Start Counter : Subsystem
  tag scope: AGC_CTRL_Capture_RSSI=global, AGC_CTRL_Capture_V_DB=global, AGC_CTRL_DONE=global, AGC_CTRL_En_IIR_Filt=global, AGC_CTRL_G_BB_SEL=global, AGC_CTRL_Set_G_RF=global, AGC_CTRL_Start_DCO=global, AGC_DONE_G_BB=global, AGC_DONE_G_RF=global, AGC_DONE_RXHP=global
  wires:
  Posedge0/1(Q) -> Done Generator/2(Run), Start Counter/2(Start)
  Run/1 -> Posedge0/1(D)
  Done Generator/1(Done) -> Start Counter/3(Done), Reset Counter/2(Done)
  IQ Valid/1 -> Start Counter/1(IQ Valid), Reset Counter/1(IQ Valid), Done Generator/1(IQ Valid)
  Start Counter/1(Count) -> [AGC_CTRL_CNTR]
  Reset Counter/1(Count) -> [AGC_RESET_CNTR]
  [AGC_RESET_CNTR] -> Relational6/1
  [reg_AGC_TIMING_RESET_G_RF] -> Relational6/2
  Relational6/1 -> Posedge9/1(D)
  [AGC_RESET_CNTR] -> Relational4/1
  [reg_AGC_TIMING_RESET_G_BB] -> Relational4/2
  Relational4/1 -> Posedge8/1(D)
  [AGC_RESET_CNTR] -> Relational3/1
  [reg_AGC_TIMING_RESET_RXHP] -> Relational3/2
  Relational3/1 -> Posedge7/1(D)
  Relational/1 -> Posedge1/1(D)
  Posedge1/1(Q) -> Logical3/1, Delay1/1
  [reg_AGC_TIMING_CAPT_RSSI_1] -> Relational/2
  Relational1/1 -> Posedge3/1(D)
  Posedge3/1(Q) -> [AGC_CTRL_Capture_V_DB], Delay/1
  [reg_AGC_TIMING_CAPT_V_DB] -> Relational1/2
  [AGC_CTRL_CNTR] -> Relational/1
  [AGC_CTRL_CNTR] -> Relational1/1
  Counter1/1 -> [AGC_CTRL_G_BB_SEL]
  Logical2/1 -> Counter1/2
  [AGC_CTRL_CNTR] -> Relational2/1
  [reg_AGC_TIMING_CAPT_RSSI_2] -> Relational2/2
  Relational2/1 -> Posedge2/1(D)
  Posedge2/1(Q) -> Logical3/2, Delay2/1
  Logical3/1 -> [AGC_CTRL_Capture_RSSI]
  Delay1/1 -> [AGC_CTRL_Set_G_RF]
  Relational5/1 -> Posedge4/1(D)
  Posedge4/1(Q) -> [AGC_CTRL_Start_DCO]
  [reg_AGC_TIMING_START_DCO] -> Relational5/2
  [AGC_CTRL_CNTR] -> Relational5/1
  Relational7/1 -> Posedge5/1(D)
  Posedge5/1(Q) -> [AGC_CTRL_En_IIR_Filt]
  [reg_AGC_TIMING_EN_IIR] -> Relational7/2
  [AGC_CTRL_CNTR] -> Relational7/1
  S-R Latch/1(Q) -> Counter1/1, Delay3/1
  Relational8/1 -> Posedge6/1(D)
  Posedge6/1(Q) -> [AGC_CTRL_DONE]
  [reg_AGC_TIMING_DONE] -> Relational8/2
  [AGC_CTRL_CNTR] -> Relational8/1
  Delay/1 -> Logical2/2
  Delay2/1 -> Logical2/1
  [reg_AGC_RESET] -> Logical1/1, Logical4/1, Logical5/1
  Logical1/1 -> [AGC_DONE_RXHP]
  Logical4/1 -> [AGC_DONE_G_BB]
  Logical5/1 -> [AGC_DONE_G_RF]
  Posedge7/1(Q) -> Logical1/2
  Posedge8/1(Q) -> Logical4/2
  Posedge9/1(Q) -> Logical5/2
  [AGC_DONE_G_BB] -> S-R Latch/1(S)
  Delay3/1 -> S-R Latch/2(R)

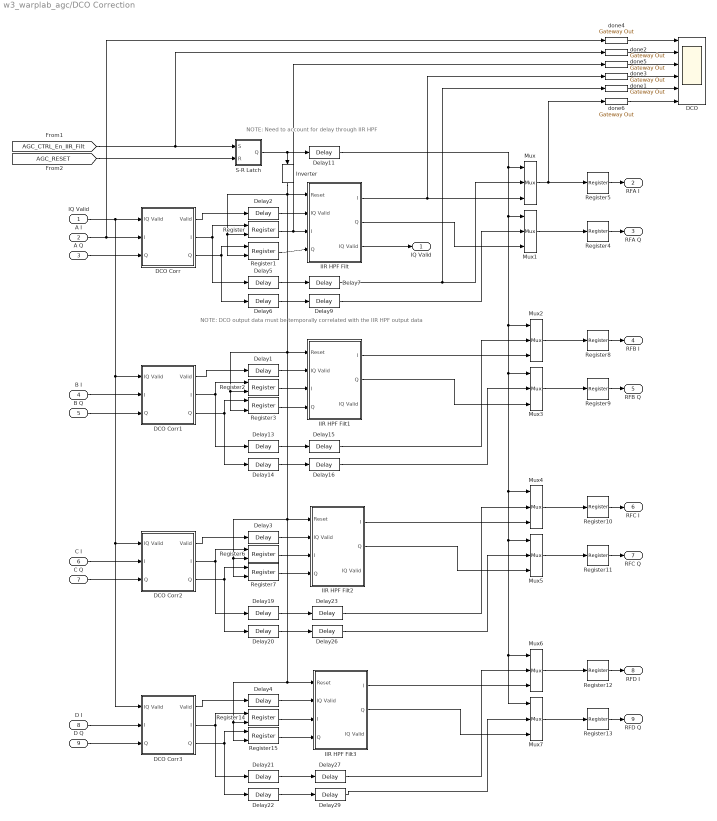
== system w3_warplab_agc/DCO Correction ==
  note: NOTE:  Need to account for
      |             delay through IIR HPF
  note: NOTE:  DCO output data must be temporally
      |            correlated with the IIR HPF output data
  IQ Valid : Inport
  A I : Inport  Port=2
  A Q : Inport  Port=3
  B I : Inport  Port=4
  B Q : Inport  Port=5
  C I : Inport  Port=6
  C Q : Inport  Port=7
  D I : Inport  Port=8
  D Q : Inport  Port=9
  DCO : Scope  NumInputPorts=6
      settings: TimeRange=10000  YMin=-1~0~-1~-1~-1~-1  YMax=1~1~1~1~1~1  SaveName=ScopeData3
  DCO Corr : Subsystem
  DCO Corr1 : Subsystem
  DCO Corr2 : Subsystem
  DCO Corr3 : Subsystem
  Delay{1..6,13..14,19..22} (12 alike) : xbsIndex_r4/Delay  rst=off  infoeditControl=Selection of Reset will increase slice count due to use of real FFs and instead of SRLs  en=off  latency=1  dbl_ovrd=off  reg_retiming=off  block_type=delay
  Delay11 : xbsIndex_r4/Delay  rst=off  infoeditControl=Selection of Reset will increase slice count due to use of real FFs and instead of SRLs  en=off  latency=7  dbl_ovrd=off  reg_retiming=off  block_type=delay
  Delay{7,9,15..16,23,26..27,29} (8 alike) : xbsIndex_r4/Delay  rst=off  infoeditControl=Selection of Reset will increase slice count due to use of real FFs and instead of SRLs  en=off  latency=6  dbl_ovrd=off  reg_retiming=off  block_type=delay
  IIR HPF Filt : Subsystem
  IIR HPF Filt1 : Subsystem
  IIR HPF Filt2 : Subsystem
  IIR HPF Filt3 : Subsystem
  Inverter : xbsIndex_r4/Inverter  en=off  latency=0  dbl_ovrd=off  block_type=inv
  Mux{,1..7} (8 alike) : xbsIndex_r4/Mux  inputs=2  en=off  latency=0  precision=Full  arith_type=Unsigned  n_bits=16  bin_pt=14  quantization=Truncate  overflow=Wrap  dbl_ovrd=off  block_type=mux
  Register{,1..3,6..7,14..15} (8 alike) : xbsIndex_r4/Register  init=0  rst=on  en=off  dbl_ovrd=off  block_type=register
  Register{4..5,8..13} (8 alike) : xbsIndex_r4/Register  init=0  rst=off  en=off  dbl_ovrd=off  block_type=register
  S-R Latch : Subsystem
  done{1..6} (6 alike) : xbsIndex_r4/Gateway Out  inherit_from_input=off  hdl_port=off  timing_constraint=None  locs_specified=off  LOCs={}  UseAsDAC=off  DACChannel='1'  block_type=gatewayout
      settings: infoedit="Gateway out block.  Converts Xilinx fixed point inputs into ouputs of type Simulink integer, double, or fixed point.<P><P>Hardware notes:  In hardware these blocks become top level output ports or are discarded, depending on how they are configured."  xl_area=[0 0 0 0 1 0 0]  block_version=VER_STRING_GOES_HERE
  " IQ Valid" : Outport
  " RFA I" : Outport  Port=2
  " RFA Q" : Outport  Port=3
  RFB I : Outport  Port=4
  RFB Q : Outport  Port=5
  RFC I : Outport  Port=6
  RFC Q : Outport  Port=7
  RFD I : Outport  Port=8
  RFD Q : Outport  Port=9
  wires:
  IIR HPF Filt/2(" Q") -> Mux1/3
  IIR HPF Filt/3(" IQ Valid") -> " IQ Valid"/1
  [AGC_CTRL_En_IIR_Filt] -> S-R Latch/1(S), done2/1
  [AGC_RESET] -> S-R Latch/2(R)
  IQ Valid/1 -> DCO Corr/1(IQ Valid), DCO Corr1/1(IQ Valid), DCO Corr2/1(IQ Valid), DCO Corr3/1(IQ Valid)
  A I/1 -> DCO Corr/2(I), done4/1
  A Q/1 -> DCO Corr/3(Q)
  IIR HPF Filt/1(" I") -> Mux/3, done3/1
  Mux/1 -> done6/1, Register5/1
  Mux1/1 -> Register4/1
  S-R Latch/1(Q) -> Inverter/1, Delay11/1
  DCO Corr/2(" I") -> Register/1, Delay5/1
  DCO Corr/3(" Q") -> Register1/1, Delay6/1
  Inverter/1 -> Register/2, Register1/2, IIR HPF Filt/1(Reset), IIR HPF Filt1/1(Reset), Register2/2, Register3/2, IIR HPF Filt2/1(Reset), IIR HPF Filt3/1(Reset), Register14/2, Register15/2, Register6/2, Register7/2
  DCO Corr/1(Valid) -> Delay2/1
  Delay2/1 -> IIR HPF Filt/2(IQ Valid)
  Register/1 -> IIR HPF Filt/3(I), done5/1
  Register1/1 -> IIR HPF Filt/4(Q)
  done4/1 -> DCO/1
  done2/1 -> DCO/2
  done5/1 -> DCO/3
  done3/1 -> DCO/4
  IIR HPF Filt1/2(" Q") -> Mux3/3
  IIR HPF Filt1/1(" I") -> Mux2/3
  DCO Corr1/2(" I") -> Delay13/1, Register2/1
  DCO Corr1/3(" Q") -> Delay14/1, Register3/1
  Delay1/1 -> IIR HPF Filt1/2(IQ Valid)
  Register2/1 -> IIR HPF Filt1/3(I)
  Register3/1 -> IIR HPF Filt1/4(Q)
  Mux2/1 -> Register8/1
  Mux3/1 -> Register9/1
  B Q/1 -> DCO Corr1/3(Q)
  B I/1 -> DCO Corr1/2(I)
  Register5/1 -> " RFA I"/1
  Register8/1 -> RFB I/1
  Register9/1 -> RFB Q/1
  Register4/1 -> " RFA Q"/1
  IIR HPF Filt2/2(" Q") -> Mux5/3
  IIR HPF Filt2/1(" I") -> Mux4/3
  DCO Corr2/2(" I") -> Delay19/1, Register6/1
  DCO Corr2/3(" Q") -> Delay20/1, Register7/1
  DCO Corr2/1(Valid) -> Delay3/1
  Delay3/1 -> IIR HPF Filt2/2(IQ Valid)
  Register6/1 -> IIR HPF Filt2/3(I)
  Register7/1 -> IIR HPF Filt2/4(Q)
  Mux4/1 -> Register10/1
  Mux5/1 -> Register11/1
  C Q/1 -> DCO Corr2/3(Q)
  C I/1 -> DCO Corr2/2(I)
  Register10/1 -> RFC I/1
  Register11/1 -> RFC Q/1
  IIR HPF Filt3/2(" Q") -> Mux7/3
  IIR HPF Filt3/1(" I") -> Mux6/3
  DCO Corr3/2(" I") -> Delay21/1, Register14/1
  DCO Corr3/3(" Q") -> Delay22/1, Register15/1
  DCO Corr3/1(Valid) -> Delay4/1
  Delay4/1 -> IIR HPF Filt3/2(IQ Valid)
  Register14/1 -> IIR HPF Filt3/3(I)
  Register15/1 -> IIR HPF Filt3/4(Q)
  Mux6/1 -> Register12/1
  Mux7/1 -> Register13/1
  D Q/1 -> DCO Corr3/3(Q)
  D I/1 -> DCO Corr3/2(I)
  Register12/1 -> RFD I/1
  Register13/1 -> RFD Q/1
  Delay5/1 -> Delay7/1
  Delay6/1 -> Delay9/1
  Delay7/1 -> Mux/2, done1/1
  Delay9/1 -> Mux1/2
  Delay11/1 -> Mux/1, Mux1/1, Mux2/1, Mux3/1, Mux4/1, Mux5/1, Mux6/1, Mux7/1
  Delay13/1 -> Delay15/1
  Delay14/1 -> Delay16/1
  Delay15/1 -> Mux2/2
  Delay16/1 -> Mux3/2
  Delay19/1 -> Delay23/1
  Delay20/1 -> Delay26/1
  Delay21/1 -> Delay27/1
  Delay22/1 -> Delay29/1
  Delay23/1 -> Mux4/2
  Delay26/1 -> Mux5/2
  Delay27/1 -> Mux6/2
  Delay29/1 -> Mux7/2
  DCO Corr1/1(Valid) -> Delay1/1
  done1/1 -> DCO/5
  done6/1 -> DCO/6
